simulink model "termic"  (Simulink 7.2)
settings: Solver=ode45  StartTime=0.0  StopTime=7000.0  RelTol=1e-3
values from neighbouring files (symbols this model uses):
  T = 800    [koef.m]
settings Model: Creator=dpara  LastModifiedBy=dpara

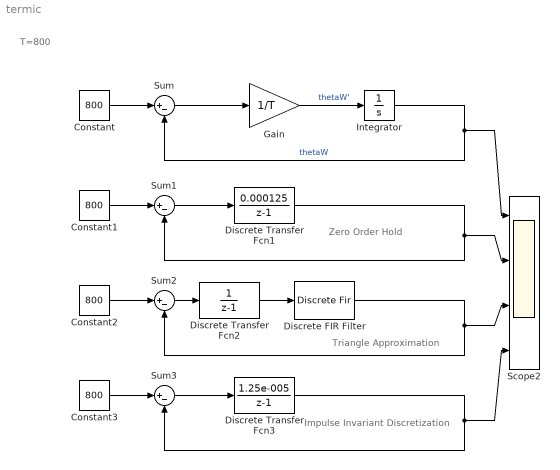
== system termic ==
  note: T=800
  note: Zero Order Hold
  note: Triangle Approximation
  note: Impulse Invariant Discretization
  Constant{,1..3} (4 alike) : Constant  Value=800  OutDataType=sfix(16)  OutScaling=2^0
  Discrete Transfer Fcn1 : DiscreteTransferFcn  Numerator=[0.000125]  Denominator=[1 -1]  SampleTime=0.1
  Discrete Transfer Fcn2 : DiscreteTransferFcn  Denominator=[1 -1]  SampleTime=0.1
  Discrete Transfer Fcn3 : DiscreteTransferFcn  Numerator=[1.25e-005]  Denominator=[1 -1]  SampleTime=0.01
  Discrete FIR Filter : DiscreteFir  NumCoeffs=[6.25e-005 6.25e-005]  SampleTime=0.1
  Gain : Gain  Gain=1/T  ParameterDataType=sfix(16)  ParameterScaling=2^0  OutDataType=sfix(16)  OutScaling=2^0
  Integrator : Integrator  InitialCondition=20
  Scope2 : Scope  NumInputPorts=4
      settings: TimeRange=7000  YMin=0~0~-5~-5  YMax=800~800~5~5  SampleInput=on  SampleTime=1
  Sum{,1..3} (4 alike) : Sum  Inputs=|+-  OutDataType=sfix(16)  OutScaling=2^0
  wires:
  Constant/1 -> Sum/1
  Sum/1 -> Gain/1
  Integrator/1 -> Sum/2, Scope2/1  "thetaW"
  Gain/1 -> Integrator/1  "thetaW'"
  Constant1/1 -> Sum1/1
  Sum1/1 -> Discrete Transfer Fcn1/1
  Discrete Transfer Fcn1/1 -> Sum1/2, Scope2/2
  Constant2/1 -> Sum2/1
  Sum2/1 -> Discrete Transfer Fcn2/1
  Discrete FIR Filter/1 -> Sum2/2, Scope2/3
  Constant3/1 -> Sum3/1
  Sum3/1 -> Discrete Transfer Fcn3/1
  Discrete Transfer Fcn3/1 -> Sum3/2, Scope2/4
  Discrete Transfer Fcn2/1 -> Discrete FIR Filter/1
